simulink model "evtol_vehicle_fmu"  (R2024a)
settings: Solver=ode4  StartTime=0.0  StopTime=1  FixedStep=0.01  RelTol=1e-3
libraries: simulink_extras x3, sharedtransform x2
settings Model: Creator=cma  LastModifiedBy=Leo.Wong
settings DataIOCC: SaveOutput=off
settings OptimizationCC: ReuseModelBlockBuffer=off
settings RTWCC: GenCodeOnly=on  GPUComputeCapability=3.5

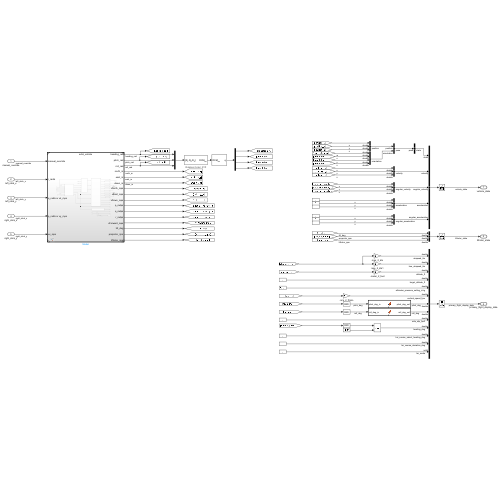
[thumbnail: Simulink's stored preview of the top-level diagram]
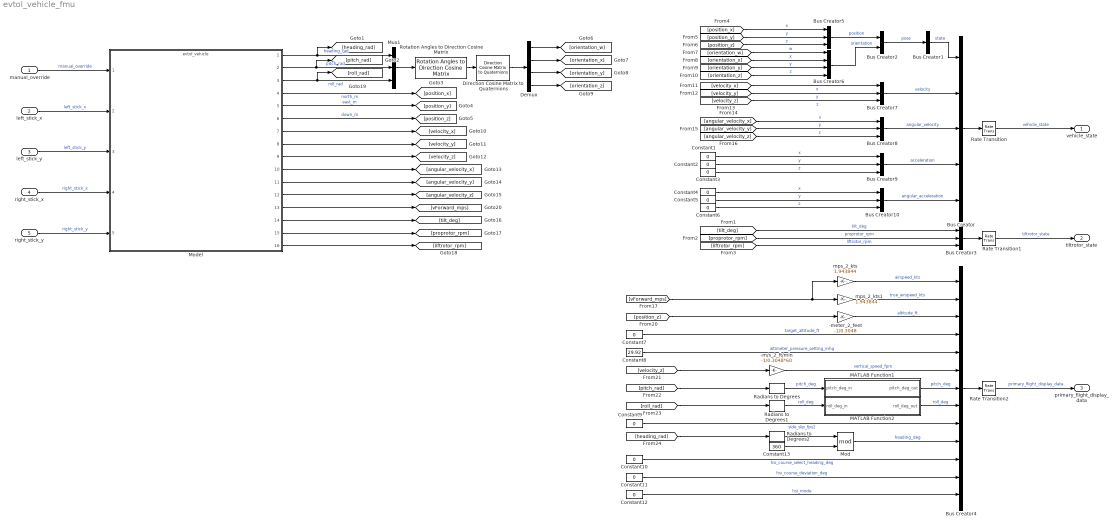
== system evtol_vehicle_fmu ==
  manual_override : Inport
  left_stick_x : Inport  Port=2
  left_stick_y : Inport  Port=3
  right_stick_x : Inport  Port=4
  right_stick_y : Inport  Port=5
  -m/s_2_ft/min : Gain  Gain=-1/0.3048*60
  -meter_2_feet : Gain  Gain=-1/0.3048
  Bus Creator : BusCreator  Inputs=5  OutDataTypeStr=Bus: vehicle_state
  Bus Creator1 : BusCreator  Inputs=1  OutDataTypeStr=Bus: state
  Bus Creator10 : BusCreator  Inputs=3  OutDataTypeStr=Bus: angular_acceleration
  Bus Creator2 : BusCreator  Inputs=2  OutDataTypeStr=Bus: pose
  Bus Creator3 : BusCreator  Inputs=3  OutDataTypeStr=Bus: tiltrotor_state
  Bus Creator4 : BusCreator  Inputs=13  OutDataTypeStr=Bus: primary_flight_display_data
  Bus Creator5 : BusCreator  Inputs=3  OutDataTypeStr=Bus: position
  Bus Creator6 : BusCreator  Inputs=4  OutDataTypeStr=Bus: orientation
  Bus Creator7 : BusCreator  Inputs=3  OutDataTypeStr=Bus: velocity
  Bus Creator8 : BusCreator  Inputs=3  OutDataTypeStr=Bus: angular_velocity
  Bus Creator9 : BusCreator  Inputs=3  OutDataTypeStr=Bus: acceleration
  Constant{1..7,9..11} (10 alike) : Constant  Value=0  OutDataTypeStr=double
  Constant12 : Constant  Value=0  OutDataTypeStr=int64
  Constant13 : Constant  Value=360  OutDataTypeStr=double
  Constant8 : Constant  Value=29.92  OutDataTypeStr=double
  Demux : Demux
  Direction Cosine Matrix to Quaternions : sharedtransform/Direction Cosine Matrix  to Quaternions  aMode=0  action=None  tolerance=eps(2)
      settings: LibrarySourceBlock=|
      | aerolibtransform2/Direction Cosine Matrix
      | to Quaternions
  MATLAB Function1 : MATLAB Function  TreatAsAtomicUnit=on
  MATLAB Function2 : MATLAB Function  TreatAsAtomicUnit=on
  Mod : Math  Operator=mod
  Model : ModelReference  ModelNameDialog=evtol_vehicle.slx  SimulationMode=Normal  ModelReferenceVersion=4.92
  Mux1 : Mux  Inputs=3
  Radians to Degrees : simulink_extras/Transformations/Radians to Degrees
  Radians to Degrees1 : simulink_extras/Transformations/Radians to Degrees
  Radians to Degrees2 : simulink_extras/Transformations/Radians to Degrees
  Rate Transition : RateTransition  OutPortSampleTime=0.01
  Rate Transition1 : RateTransition  OutPortSampleTime=0.01
  Rate Transition2 : RateTransition  OutPortSampleTime=0.01
  Rotation Angles to Direction Cosine Matrix : sharedtransform/Rotation Angles to Direction Cosine Matrix  rotationOrder=XYZ  aMode=aMode
  mps_2_kts : Gain  Gain=1.943844
  mps_2_kts1 : Gain  Gain=1.943844
  vehicle_state : Outport  OutDataTypeStr=Bus: vehicle_state
  tiltrotor_state : Outport  Port=2  OutDataTypeStr=Bus: tiltrotor_state
  primary_flight_display_data : Outport  Port=3  OutDataTypeStr=Bus: primary_flight_display_data
  wires:
  Model/5 -> [position_y]  "east_m"
  Model/6 -> [position_z]  "down_m"
  Model/4 -> [position_x]  "north_m"
  Direction Cosine Matrix to Quaternions/1 -> Demux/1
  Rotation Angles to Direction Cosine Matrix/1 -> Direction Cosine Matrix to Quaternions/1
  Mux1/1 -> Rotation Angles to Direction Cosine Matrix/1
  Demux/1 -> [orientation_w]
  Model/7 -> [velocity_x]
  Model/8 -> [velocity_y]
  Model/9 -> [velocity_z]
  Model/10 -> [angular_velocity_x]
  Model/11 -> [angular_velocity_y]
  Model/12 -> [angular_velocity_z]
  Bus Creator/1 -> Rate Transition/1
  Bus Creator1/1 -> Bus Creator/1  "state"
  Bus Creator2/1 -> Bus Creator1/1  "pose"
  [position_x] -> Bus Creator5/1  "x"
  [position_y] -> Bus Creator5/2  "y"
  [position_z] -> Bus Creator5/3  "z"
  [orientation_w] -> Bus Creator6/1  "w"
  [orientation_x] -> Bus Creator6/2  "x"
  [orientation_y] -> Bus Creator6/3  "y"
  [orientation_z] -> Bus Creator6/4  "z"
  Bus Creator7/1 -> Bus Creator/2  "velocity"
  Bus Creator8/1 -> Bus Creator/3  "angular_velocity"
  [velocity_x] -> Bus Creator7/1  "x"
  [velocity_y] -> Bus Creator7/2  "y"
  [velocity_z] -> Bus Creator7/3  "z"
  [angular_velocity_x] -> Bus Creator8/1  "x"
  [angular_velocity_y] -> Bus Creator8/2  "y"
  [angular_velocity_z] -> Bus Creator8/3  "z"
  Bus Creator9/1 -> Bus Creator/4  "acceleration"
  Bus Creator10/1 -> Bus Creator/5  "angular_acceleration"
  Constant1/1 -> Bus Creator9/1  "x"
  Constant2/1 -> Bus Creator9/2  "y"
  Constant3/1 -> Bus Creator9/3  "z"
  Constant4/1 -> Bus Creator10/1  "x"
  Constant5/1 -> Bus Creator10/2  "y"
  Constant6/1 -> Bus Creator10/3  "z"
  Rate Transition/1 -> vehicle_state/1  "vehicle_state"
  Demux/2 -> [orientation_x]
  Demux/3 -> [orientation_y]
  Demux/4 -> [orientation_z]
  Model/1 -> [heading_rad], Mux1/1  "heading_rad"
  Model/2 -> [pitch_rad], Mux1/2  "pitch_rad"
  Model/3 -> [roll_rad], Mux1/3  "roll_rad"
  right_stick_y/1 -> Model/5  "right_stick_y"
  right_stick_x/1 -> Model/4  "right_stick_x"
  left_stick_y/1 -> Model/3  "left_stick_y"
  left_stick_x/1 -> Model/2  "left_stick_x"
  manual_override/1 -> Model/1  "manual_override"
  Bus Creator5/1 -> Bus Creator2/1  "position"
  Bus Creator6/1 -> Bus Creator2/2  "orientation"
  Bus Creator3/1 -> Rate Transition1/1
  [tilt_deg] -> Bus Creator3/1  "tilt_deg"
  [proprotor_rpm] -> Bus Creator3/2  "proprotor_rpm"
  [liftrotor_rpm] -> Bus Creator3/3  "liftrotor_rpm"
  Rate Transition1/1 -> tiltrotor_state/1  "tiltrotor_state"
  Rate Transition2/1 -> primary_flight_display_data/1  "primary_flight_display_data"
  Bus Creator4/1 -> Rate Transition2/1
  [vForward_mps] -> mps_2_kts/1, mps_2_kts1/1
  mps_2_kts/1 -> Bus Creator4/1  "airspeed_kts"
  mps_2_kts1/1 -> Bus Creator4/2  "true_airspeed_kts"
  -meter_2_feet/1 -> Bus Creator4/3  "altitude_ft"
  [position_z] -> -meter_2_feet/1
  Constant7/1 -> Bus Creator4/4  "target_altitude_ft"
  Constant8/1 -> Bus Creator4/5  "altimeter_pressure_setting_inhg"
  [velocity_z] -> -m/s_2_ft/min/1
  Radians to Degrees/1 -> MATLAB Function1/1(pitch_deg_in)  "pitch_deg"
  [pitch_rad] -> Radians to Degrees/1
  Radians to Degrees1/1 -> MATLAB Function2/1(roll_deg_in)  "roll_deg"
  [roll_rad] -> Radians to Degrees1/1
  Constant9/1 -> Bus Creator4/9  "side_slip_fps2"
  [heading_rad] -> Radians to Degrees2/1
  Constant10/1 -> Bus Creator4/11  "hsi_course_select_heading_deg"
  Constant11/1 -> Bus Creator4/12  "hsi_course_deviation_deg"
  Constant12/1 -> Bus Creator4/13  "hsi_mode"
  Mod/1 -> Bus Creator4/10  "heading_deg"
  Constant13/1 -> Mod/2
  Radians to Degrees2/1 -> Mod/1
  MATLAB Function1/1(pitch_deg_out) -> Bus Creator4/7  "pitch_deg"
  MATLAB Function2/1(roll_deg_out) -> Bus Creator4/8  "roll_deg"
  -m/s_2_ft/min/1 -> Bus Creator4/6  "vertical_speed_fpm"
  Model/13 -> [vForward_mps]
  Model/14 -> [tilt_deg]
  Model/15 -> [proprotor_rpm]
  Model/16 -> [liftrotor_rpm]

== matlab function evtol_vehicle_fmu/MATLAB Function2 ==
  data: roll_deg_in input; roll_deg_out output
function roll_deg_out = fcn(roll_deg_in)

roll_deg_out = mod(roll_deg_in, 360);
if roll_deg_out > 180
    roll_deg_out = roll_deg_out - 360;
end

== matlab function evtol_vehicle_fmu/MATLAB Function1 ==
  data: pitch_deg_in input; pitch_deg_out output
function pitch_deg_out = fcn(pitch_deg_in)

pitch_deg_in = mod(pitch_deg_in, 360);
if pitch_deg_in >= 0 && pitch_deg_in <= 90
    pitch_deg_out = pitch_deg_in;
elseif pitch_deg_in > 90 && pitch_deg_in < 180
    pitch_deg_out = 90 - mod(pitch_deg_in, 90);
elseif pitch_deg_in >= 180 && pitch_deg_in <= 270
    pitch_deg_out = 180 - pitch_deg_in;
elseif pitch_deg_in > 270
    pitch_deg_out = pitch_deg_in - 360;
else
    pitch_deg_out = pitch_deg_in;
end
